simulink model "model_task2"  (R2022b)
settings: Solver=FixedStepAuto  StartTime=0.0  StopTime=10  FixedStep=0.1  RelTol=1e-3
settings Model: Creator=anton  LastModifiedBy=anton

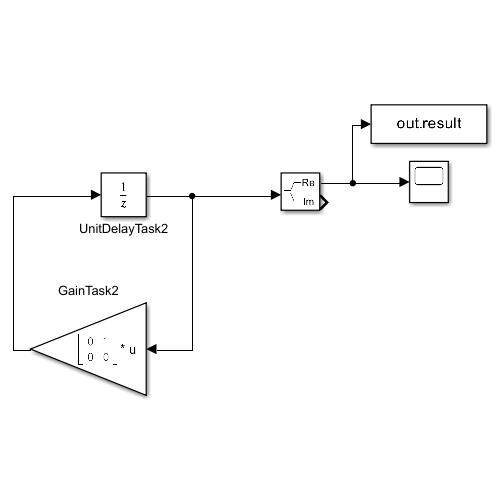
[thumbnail: Simulink's stored preview of the top-level diagram]
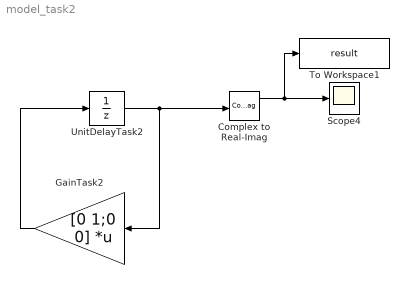
== system model_task2 ==
  Complex to Real-Imag : ComplexToRealImag
  GainTask2 : Gain  Gain=[0 1;0 0]  Multiplication=Matrix(K*u)
  Scope4 : Scope
  To Workspace1 : ToWorkspace  VariableName=result  SaveFormat=Timeseries  SampleTime=-1
  UnitDelayTask2 : UnitDelay  InitialCondition=[5;-3]  SampleTime=-1  HasFrameUpgradeWarning=on
  wires:
  GainTask2/1 -> UnitDelayTask2/1
  UnitDelayTask2/1 -> GainTask2/1, Complex to Real-Imag/1
  Complex to Real-Imag/1 -> To Workspace1/1, Scope4/1
